simulink model "MuscleGeometry"  (R2024b)
settings: Solver=VariableStepAuto  StartTime=0.0  StopTime=10.0  RelTol=1e-3
undefined symbols (not defined in the file or in its folder): L2, M_BICB, M_BRACH, M_TRIPB
settings Model: Creator=jakub  LastModifiedBy=jakub

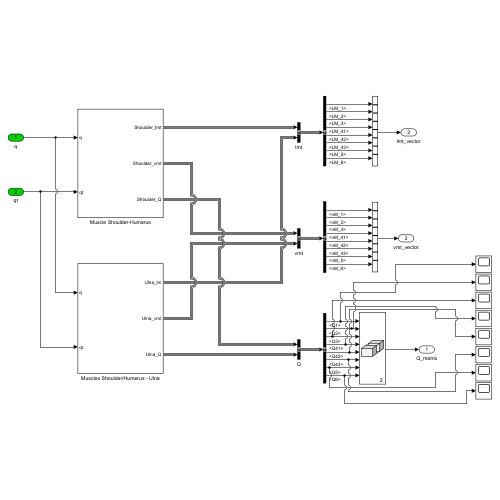
[thumbnail: Simulink's stored preview of the top-level diagram]
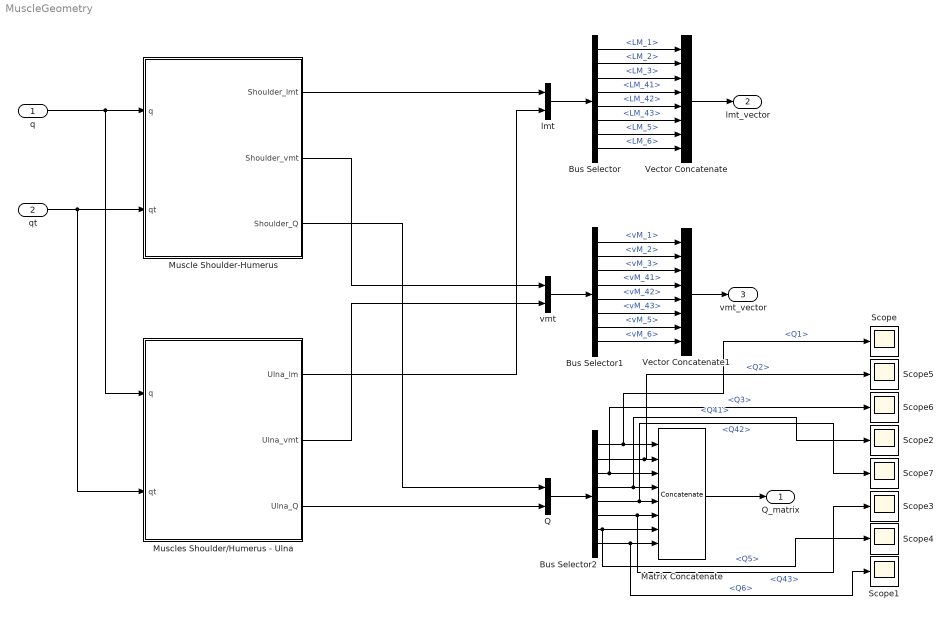
== system MuscleGeometry ==
  q : Inport  OutDataTypeStr=double  Unit=rad  PortDimensions=[2 1]  SampleTime=0
  qt : Inport  Port=2  OutDataTypeStr=double  Unit=rad/sec  PortDimensions=[2 1]  SampleTime=0
  Bus Selector : BusSelector  OutputSignals=signal1.LM_1,signal1.LM_2,signal1.LM_3,signal2.LM_41,signal2.LM_42,signal2.LM_43,signal2.LM_5,signal2.LM_6
  Bus Selector1 : BusSelector  OutputSignals=signal1.vM_1,signal1.vM_2,signal1.vM_3,signal2.vM_41,signal2.vM_42,signal2.vM_43,signal2.vM_5,signal2.vM_6
  Bus Selector2 : BusSelector  OutputSignals=signal1.Q1,signal1.Q2,signal1.Q3,signal2.Q41,signal2.Q42,signal2.Q43,signal2.Q5,signal2.Q6
  Matrix Concatenate : Concatenate  NumInputs=8  Mode=Multidimensional array  ConcatenateDimension=2
  Muscle Shoulder-Humerus : Subsystem
  Muscles Shoulder/Humerus - Ulna : Subsystem
  Q : BusCreator  Inputs=2
  Scope{,1..7} (8 alike) : Scope
  Vector Concatenate : Concatenate  NumInputs=8
  Vector Concatenate1 : Concatenate  NumInputs=8
  lmt : BusCreator  Inputs=2
  vmt : BusCreator  Inputs=2
  Q_matrix : Outport  OutDataTypeStr=double  PortDimensions=[2 8]  SampleTime=0
  lmt_vector : Outport  Port=2  OutDataTypeStr=double  Unit=m  PortDimensions=8  SampleTime=0
  vmt_vector : Outport  Port=3  OutDataTypeStr=double  Unit=m/s  PortDimensions=8  SampleTime=0
  wires:
  q/1 -> Muscle Shoulder-Humerus/1(q), Muscles Shoulder/Humerus - Ulna/1(q)
  qt/1 -> Muscle Shoulder-Humerus/2(qt), Muscles Shoulder/Humerus - Ulna/2(qt)
  Muscle Shoulder-Humerus/1(Shoulder_lmt) -> lmt/1
  Muscles Shoulder/Humerus - Ulna/1(Ulna_lm) -> lmt/2
  Muscle Shoulder-Humerus/2(Shoulder_vmt) -> vmt/1
  Muscles Shoulder/Humerus - Ulna/2(Ulna_vmt) -> vmt/2
  Muscle Shoulder-Humerus/3(Shoulder_Q) -> Q/1
  Muscles Shoulder/Humerus - Ulna/3(Ulna_Q) -> Q/2
  lmt/1 -> Bus Selector/1
  Bus Selector/1 -> Vector Concatenate/1  "<LM_1>"
  Bus Selector/2 -> Vector Concatenate/2  "<LM_2>"
  Bus Selector/3 -> Vector Concatenate/3  "<LM_3>"
  Bus Selector/4 -> Vector Concatenate/4  "<LM_41>"
  Bus Selector/5 -> Vector Concatenate/5  "<LM_42>"
  Bus Selector/6 -> Vector Concatenate/6  "<LM_43>"
  Bus Selector/7 -> Vector Concatenate/7  "<LM_5>"
  Bus Selector/8 -> Vector Concatenate/8  "<LM_6>"
  Vector Concatenate/1 -> lmt_vector/1
  vmt/1 -> Bus Selector1/1
  Bus Selector1/1 -> Vector Concatenate1/1  "<vM_1>"
  Bus Selector1/2 -> Vector Concatenate1/2  "<vM_2>"
  Bus Selector1/3 -> Vector Concatenate1/3  "<vM_3>"
  Bus Selector1/4 -> Vector Concatenate1/4  "<vM_41>"
  Bus Selector1/5 -> Vector Concatenate1/5  "<vM_42>"
  Bus Selector1/6 -> Vector Concatenate1/6  "<vM_43>"
  Bus Selector1/7 -> Vector Concatenate1/7  "<vM_5>"
  Bus Selector1/8 -> Vector Concatenate1/8  "<vM_6>"
  Q/1 -> Bus Selector2/1
  Bus Selector2/1 -> Scope/1, Matrix Concatenate/1  "<Q1>"
  Bus Selector2/2 -> Scope5/1, Matrix Concatenate/2  "<Q2>"
  Bus Selector2/3 -> Scope6/1, Matrix Concatenate/3  "<Q3>"
  Bus Selector2/4 -> Scope2/1, Matrix Concatenate/4  "<Q41>"
  Bus Selector2/5 -> Scope7/1, Matrix Concatenate/5  "<Q42>"
  Bus Selector2/6 -> Scope3/1, Matrix Concatenate/6  "<Q43>"
  Bus Selector2/7 -> Scope4/1, Matrix Concatenate/7  "<Q5>"
  Bus Selector2/8 -> Scope1/1, Matrix Concatenate/8  "<Q6>"
  Vector Concatenate1/1 -> vmt_vector/1
  Matrix Concatenate/1 -> Q_matrix/1

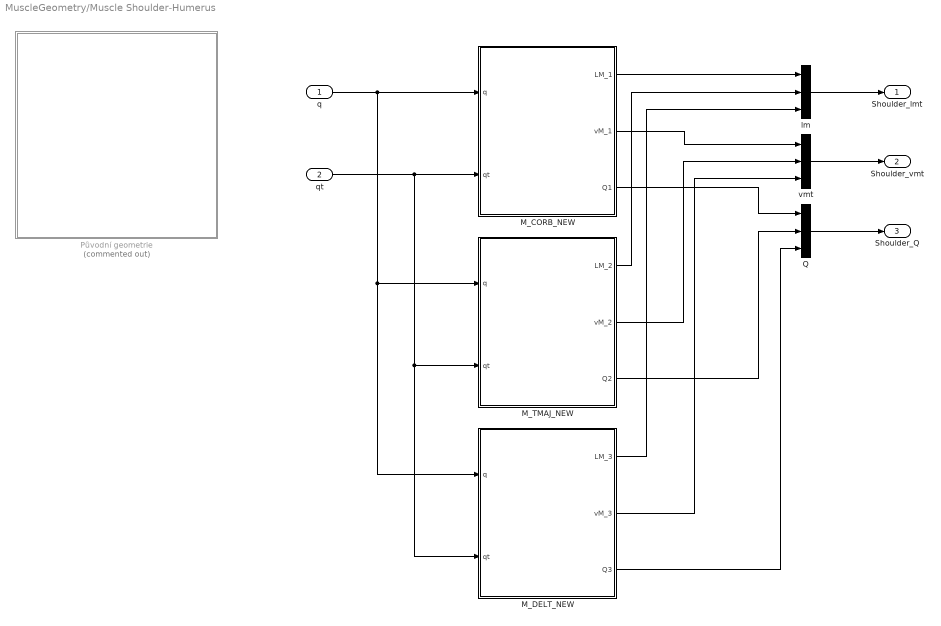
== system MuscleGeometry/Muscle Shoulder-Humerus ==
  q : Inport  OutDataTypeStr=double  Unit=rad  PortDimensions=[2 1]  SampleTime=0
  qt : Inport  Port=2  OutDataTypeStr=double  Unit=rad/sec  PortDimensions=[2 1]  SampleTime=0
  M_CORB_NEW : MATLAB Function  TreatAsAtomicUnit=on
  M_DELT_NEW : MATLAB Function  TreatAsAtomicUnit=on
  M_TMAJ_NEW : MATLAB Function  TreatAsAtomicUnit=on
  Původní geometrie : Subsystem  Commented=on
  Q : BusCreator  Inputs=3
  lm : BusCreator  Inputs=3
  vmt : BusCreator  Inputs=3
  Shoulder_lmt : Outport  OutDataTypeStr=double  Unit=m  PortDimensions=3  SampleTime=0
  Shoulder_vmt : Outport  Port=2  OutDataTypeStr=double  Unit=m/s  PortDimensions=3  SampleTime=0
  Shoulder_Q : Outport  Port=3
  wires:
  M_DELT_NEW/3(Q3) -> Q/3
  M_CORB_NEW/3(Q1) -> Q/1
  lm/1 -> Shoulder_lmt/1
  M_TMAJ_NEW/1(LM_2) -> lm/2
  vmt/1 -> Shoulder_vmt/1
  M_TMAJ_NEW/2(vM_2) -> vmt/2
  M_DELT_NEW/2(vM_3) -> vmt/3
  M_TMAJ_NEW/3(Q2) -> Q/2
  M_CORB_NEW/2(vM_1) -> vmt/1
  M_DELT_NEW/1(LM_3) -> lm/3
  M_CORB_NEW/1(LM_1) -> lm/1
  Q/1 -> Shoulder_Q/1
  qt/1 -> M_DELT_NEW/2(qt), M_TMAJ_NEW/2(qt), M_CORB_NEW/2(qt)
  q/1 -> M_CORB_NEW/1(q), M_DELT_NEW/1(q), M_TMAJ_NEW/1(q)

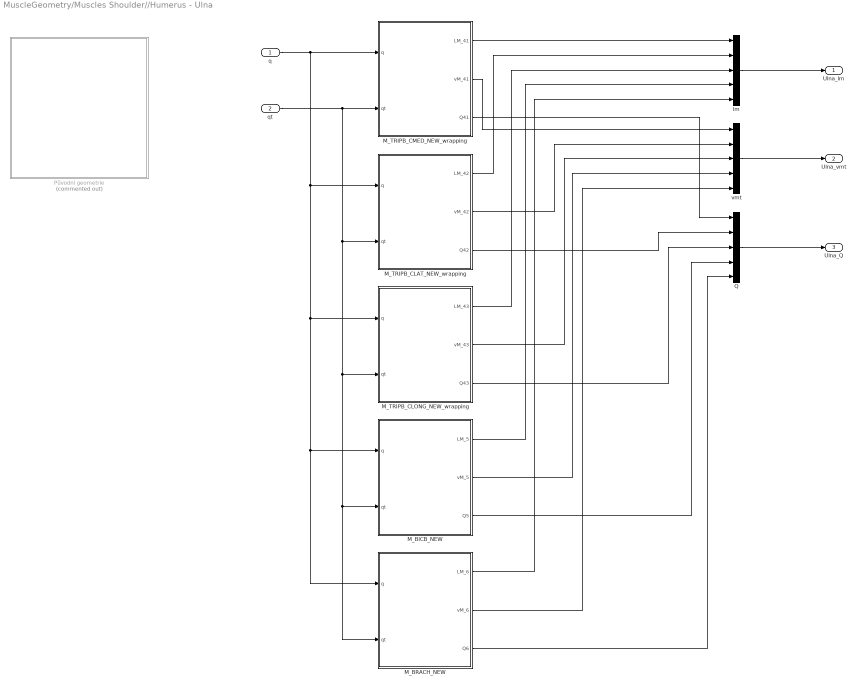
== system MuscleGeometry/Muscles Shoulder//Humerus - Ulna ==
  q : Inport  OutDataTypeStr=double  Unit=rad  PortDimensions=2  SampleTime=0
  qt : Inport  Port=2  OutDataTypeStr=double  Unit=rad/sec  PortDimensions=2  SampleTime=0
  M_BICB_NEW : MATLAB Function  TreatAsAtomicUnit=on
  M_BRACH_NEW : MATLAB Function  TreatAsAtomicUnit=on
  M_TRIPB_CLAT_NEW_wrapping : MATLAB Function  TreatAsAtomicUnit=on
  M_TRIPB_CLONG_NEW_wrapping : MATLAB Function  TreatAsAtomicUnit=on
  M_TRIPB_CMED_NEW_wrapping : MATLAB Function  TreatAsAtomicUnit=on
  Původní geometrie : Subsystem  Commented=on
  Q : BusCreator  Inputs=5
  lm : BusCreator  Inputs=5
  vmt : BusCreator  Inputs=5
  Ulna_lm : Outport
  Ulna_vmt : Outport  Port=2
  Ulna_Q : Outport  Port=3
  wires:
  M_TRIPB_CLAT_NEW_wrapping/1(LM_42) -> lm/2
  M_BRACH_NEW/1(LM_6) -> lm/5
  M_TRIPB_CMED_NEW_wrapping/1(LM_41) -> lm/1
  vmt/1 -> Ulna_vmt/1
  qt/1 -> M_TRIPB_CMED_NEW_wrapping/2(qt), M_BRACH_NEW/2(qt), M_BICB_NEW/2(qt), M_TRIPB_CLONG_NEW_wrapping/2(qt), M_TRIPB_CLAT_NEW_wrapping/2(qt)
  M_TRIPB_CLAT_NEW_wrapping/3(Q42) -> Q/2
  Q/1 -> Ulna_Q/1
  lm/1 -> Ulna_lm/1
  M_TRIPB_CMED_NEW_wrapping/2(vM_41) -> vmt/1
  M_TRIPB_CMED_NEW_wrapping/3(Q41) -> Q/1
  M_TRIPB_CLAT_NEW_wrapping/2(vM_42) -> vmt/2
  M_TRIPB_CLONG_NEW_wrapping/3(Q43) -> Q/3
  M_TRIPB_CLONG_NEW_wrapping/2(vM_43) -> vmt/3
  M_BRACH_NEW/2(vM_6) -> vmt/5
  M_BRACH_NEW/3(Q6) -> Q/5
  M_TRIPB_CLONG_NEW_wrapping/1(LM_43) -> lm/3
  M_BICB_NEW/1(LM_5) -> lm/4
  M_BICB_NEW/2(vM_5) -> vmt/4
  M_BICB_NEW/3(Q5) -> Q/4
  q/1 -> M_TRIPB_CMED_NEW_wrapping/1(q), M_BRACH_NEW/1(q), M_BICB_NEW/1(q), M_TRIPB_CLONG_NEW_wrapping/1(q), M_TRIPB_CLAT_NEW_wrapping/1(q)

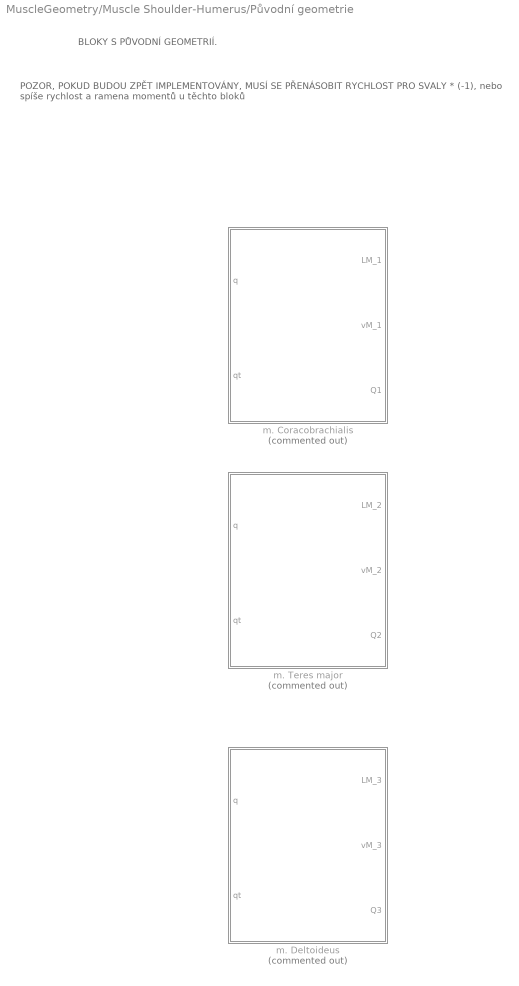
== system MuscleGeometry/Muscle Shoulder-Humerus/Původní geometrie ==
  note: POZOR, POKUD BUDOU ZPĚT IMPLEMENTOVÁNY, MUSÍ SE PŘENÁSOBIT RYCHLOST PRO SVALY * (-1), nebo spíše rychlost a ramena momentů u těchto bloků
  note: BLOKY S PŮVODNÍ GEOMETRIÍ.
  m. Coracobrachialis : MATLAB Function  Commented=on  TreatAsAtomicUnit=on
  m. Deltoideus : MATLAB Function  Commented=on  TreatAsAtomicUnit=on
  m. Teres major : MATLAB Function  Commented=on  TreatAsAtomicUnit=on

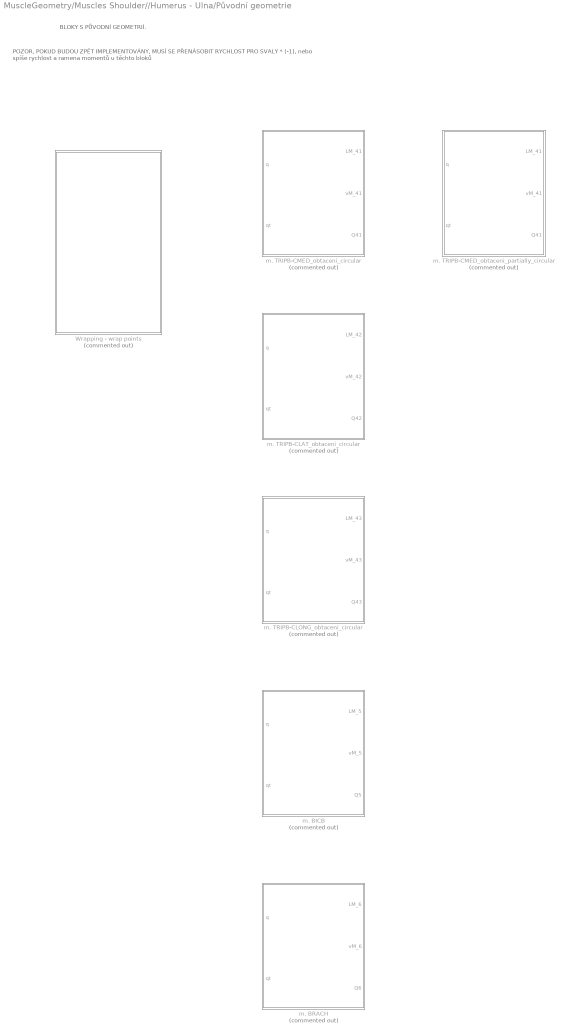
== system MuscleGeometry/Muscles Shoulder//Humerus - Ulna/Původní geometrie ==
  note: BLOKY S PŮVODNÍ GEOMETRIÍ.
  note: POZOR, POKUD BUDOU ZPĚT IMPLEMENTOVÁNY, MUSÍ SE PŘENÁSOBIT RYCHLOST PRO SVALY * (-1), nebo spíše rychlost a ramena momentů u těchto bloků
  Wrapping - wrap points : Subsystem  Commented=on
  m. BICB : MATLAB Function  Commented=on  TreatAsAtomicUnit=on
  m. BRACH : MATLAB Function  Commented=on  TreatAsAtomicUnit=on
  m. TRIPB-CLAT_obtaceni_circular : MATLAB Function  Commented=on  TreatAsAtomicUnit=on
  m. TRIPB-CLONG_obtaceni_circular : MATLAB Function  Commented=on  TreatAsAtomicUnit=on
  m. TRIPB-CMED_obtaceni_circular : MATLAB Function  Commented=on  TreatAsAtomicUnit=on
  m. TRIPB-CMED_obtaceni_partially_circular : MATLAB Function  Commented=on  TreatAsAtomicUnit=on

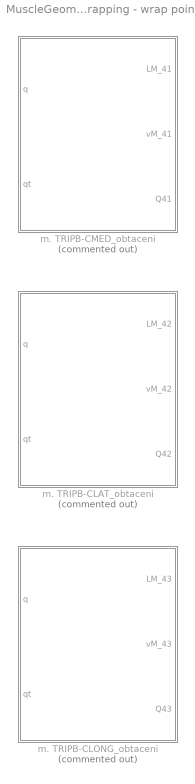
== system MuscleGeometry/Muscles Shoulder//Humerus - Ulna/Původní geometrie/Wrapping - wrap points ==
  m. TRIPB-CLAT_obtaceni : MATLAB Function  Commented=on  TreatAsAtomicUnit=on
  m. TRIPB-CLONG_obtaceni : MATLAB Function  Commented=on  TreatAsAtomicUnit=on
  m. TRIPB-CMED_obtaceni : MATLAB Function  Commented=on  TreatAsAtomicUnit=on

== matlab function MuscleGeometry/Muscles Shoulder//Humerus - Ulna/Původní geometrie/m. BICB ==
  data: LM_5 output double size=1; q input double size=[2 1]; qt input double size=[2 1]; vM_5 output double size=1; M_BICB parameter; Q5 output double size=[2 1]; L2 parameter double size=1
function [LM_5,vM_5, Q5] = MUSCLE_BICB(q,qt,M_BICB, L2)
   
    fi12 = q(1);
    fi12t = qt(1);
    fi13 = q(2);
    fi13t = qt(2);
      
     % Parameters
        % A point in local system "3"
            x3A = M_BICB.x3;
        % B point in local system "1"
            x1B = M_BICB.x1;
            y1B = M_BICB.y1;
    
    % Global coordinates of significant points    
        pA = [L2*cos(fi12) + x3A*cos(fi13);
              L2*sin(fi12) + x3A*sin(fi13)];

        pB = [x1B;
              y1B];

% OUTPUT
    % Muscle geometry
        % Length AB
            LM_5 = norm(pB-pA);

        % Unit vectors
            eAB = (pB-pA)/norm(pB-pA);

        %
            pfi12 = [ -L2*sin(fi12);
                       L2*cos(fi12)];

            pfi13 = [-x3A*sin(fi13);
                      x3A*cos(fi13)];

     % Muscle velocity


        % Final velocity in muscle
            vM_5 = dot(eAB,fi12t*pfi12 + fi13t*pfi13);

    % Vector Q - Generalized forces
        Q_1 = dot(eAB,pfi12);
        Q_2 = dot(eAB,pfi13);

        % Compact form
        Q5 = [Q_1;Q_2];
    
end

== matlab function MuscleGeometry/Muscles Shoulder//Humerus - Ulna/Původní geometrie/m. BRACH ==
  data: LM_6 output double size=1; q input double size=[2 1]; qt input double size=[2 1]; vM_6 output double size=1; M_BRACH parameter; Q6 output double size=[2 1]; L2 parameter double size=1
function [LM_6,vM_6, Q6] = MUSCLE_BRACH(q,qt,M_BRACH, L2)
   
    fi12 = q(1);
    fi12t = qt(1);
    fi13 = q(2);
    fi13t = qt(2);
    
      
     % Parameters
        % A point in local system "3"
            x3A = M_BRACH.x3;
        % B point in local system "2"
            x2B = M_BRACH.x2;

    % Global coordinates of significant points    
        pA = [L2*cos(fi12) + x3A*cos(fi13);
              L2*sin(fi12) + x3A*sin(fi13)];

        pB = [x2B*cos(fi12);
              x2B*sin(fi12)];

% OUTPUT
    % Muscle geometry
        % Length AB
            LM_6 = norm(pB-pA);

        % Unit vectors
            eAB = (pB-pA)/norm(pB-pA);

        %
            pfi12 = [ (-L2+x2B)*sin(fi12);
                       (L2-x2B)*cos(fi12)];

            pfi13 = [-x3A*sin(fi13);
                      x3A*cos(fi13)];

     % Muscle velocity


        % Final velocity in muscle
            vM_6 = dot(eAB,fi12t*pfi12 + fi13t*pfi13);

    % Vector Q - Generalized forces
        Q_1 = dot(eAB,pfi12);
        Q_2 = dot(eAB,pfi13);

        % Compact form
        Q6 = [Q_1;Q_2];
    
end

== matlab function MuscleGeometry/Muscles Shoulder//Humerus - Ulna/M_TRIPB_CMED_NEW_wrapping ==
  data: LM_41 output double size=1; q input double size=[2 1]; qt input double size=[2 1]; vM_41 output double size=1; Q41 output double size=[2 1]
function [LM_41, vM_41, Q41] = MUSCLE_TRIPB_CMED(q, qt)
% VSTUPY:
% q  = [fi12; fi13]         % Úhly
% qt = [fi12_dot; fi13_dot] % Rychlosti úhlů

    % Rozbalení vstupních proměnných
    fi12 = q(1);
    fi13 = q(2);
    fi12_dot = qt(1);
    fi13_dot = qt(2);

    % Přímé volání funkcí
    LM_41 = M_TRIPB_CMED_LM(fi12, fi13);
    vM_41 = M_TRIPB_CMED_vM(fi12, fi13, fi12_dot, fi13_dot);
    Q41 = M_TRIPB_CMED_Q(fi12, fi13);
end

== matlab function MuscleGeometry/Muscle Shoulder-Humerus/M_CORB_NEW ==
  data: LM_1 output double size=1; q input double size=[2 1]; qt input double size=[2 1]; vM_1 output double size=1; Q1 output double size=[2 1]
function [LM_1, vM_1, Q1] = MUSCLE_CORB(q, qt)
% VSTUPY:
% q  = [fi12; fi13]         % Úhly
% qt = [fi12_dot; fi13_dot] % Rychlosti úhlů

    % Rozbalení vstupních proměnných
    fi12 = q(1);
    fi12_dot = qt(1);

    % Přímé volání funkcí
    LM_1 = M_CORB_LM(fi12);
    vM_1 = M_CORB_vM(fi12, fi12_dot);
    Q1 = M_CORB_Q(fi12);
end

== matlab function MuscleGeometry/Muscle Shoulder-Humerus/M_DELT_NEW ==
  data: LM_3 output double size=1; q input double size=[2 1]; qt input double size=[2 1]; vM_3 output double size=1; Q3 output double size=[2 1]
function [LM_3, vM_3, Q3] = MUSCLE_DELT(q, qt)
% VSTUPY:
% q  = [fi12; fi13]         % Úhly
% qt = [fi12_dot; fi13_dot] % Rychlosti úhlů

    % Rozbalení vstupních proměnných
    fi12 = q(1);
    fi12_dot = qt(1);

    % Přímé volání funkcí
    LM_3 = M_DELT_LM(fi12);
    vM_3 = M_DELT_vM(fi12, fi12_dot);
    Q3 = M_DELT_Q(fi12);
end

== matlab function MuscleGeometry/Muscles Shoulder//Humerus - Ulna/Původní geometrie/m. TRIPB-CLAT_obtaceni_circular ==
  data: LM_42 output double size=1; q input double size=[2 1]; qt input double size=[2 1]; vM_42 output double size=1; M_TRIPB parameter; Q42 output double size=[2 1]; L2 parameter double size=1
function [LM_42,vM_42, Q42] = MUSCLE_TRIPB_CLAT(q,qt,M_TRIPB, L2)
   
    fi12 = q(1);
    fi12t = qt(1);
    fi13 = q(2);
    fi13t = qt(2);
      
      % Parameters
        % A point in local system "3"
            x3A = M_TRIPB.CLAT.x3;
            y3A = M_TRIPB.CLAT.y3;
        % B point in local system "2"
            x2B = M_TRIPB.CLAT.x2;
            y2B = M_TRIPB.CLAT.y2;

        % Wrapping points
            % W2 - humerus
                x2W2 = M_TRIPB.CLAT.x2W2;
                y2W2 = M_TRIPB.CLAT.y2W2;
            % W3 - ulna radius
                x3W3 = M_TRIPB.CLAT.x3W3;
                y3W3 = M_TRIPB.CLAT.y3W3;

                
    
    % Global coordinates of significant points    
        pA = [L2*cos(fi12) + x3A*cos(fi13) - y3A*sin(fi13);
              L2*sin(fi12) + x3A*sin(fi13) + y3A*cos(fi13)];

        pW3 = [L2*cos(fi12) + x3W3*cos(fi13) - y3W3*sin(fi13);
               L2*sin(fi12) + x3W3*sin(fi13) + y3W3*cos(fi13)];

        pW2 = [x2W2*cos(fi12) - y2W2*sin(fi12);
               x2W2*sin(fi12) + y2W2*cos(fi12)];

        pB = [x2B*cos(fi12) - y2B*sin(fi12);
              x2B*sin(fi12) + y2B*cos(fi12)];

% OUTPUT
    % Muscle geometry
        % Length AB
            LM_42_straight = norm(pW2-pB) + norm(pW3-pA);
            LM_42_circ = norm(pW3-pW2);
            LM_42 = LM_42_straight + LM_42_circ;

        % Unit vectors
            eAW3 = (pW3-pA)/norm(pW3-pA);
            eW3W2 = (pW2-pW3)/norm(pW2-pW3);
            eBW2 = (pW2-pB)/norm(pW2-pB);

        %
            pAfi12 = [-L2*sin(fi12);
                       L2*cos(fi12)];

            pAfi13 = [-x3A*sin(fi13) - y3A*cos(fi13);
                       x3A*cos(fi13) - y3A*sin(fi13)];

            pW3fi12 = [-L2*sin(fi12);
                        L2*cos(fi12)];

            pW3fi13 = [-x3W3*sin(fi13) - y3W3*cos(fi13);
                        x3W3*cos(fi13) - y3W3*sin(fi13)];

            pW2fi12 = [-x2W2*sin(fi12) - y2W2*cos(fi12);
                        x2W2*cos(fi12) - y2W2*sin(fi12)];
            
            pBfi12 = [-x2B*sin(fi12) - y2B*cos(fi12);
                       x2B*cos(fi12) - y2B*sin(fi12)];

     % Muscle velocity


        % Final velocity in muscle
            vM_42 = dot(eAW3,fi12t*(pAfi12 - pW3fi12) + fi13t*(pAfi13-pW3fi13)) + dot(eW3W2,fi12t*(pW3fi12-pW2fi12) + fi13t*pW3fi13) + dot(eBW2,fi12t*(-pW2fi12 + pBfi12));

    % Vector Q - Generalized forces
        Q_1 = dot(eAW3,pAfi12-pW3fi12) + dot(eW3W2,pW3fi12-pW2fi12) + dot(eBW2,-pW2fi12+pBfi12);
        Q_2 = dot(eAW3,pAfi13-pW3fi13) + dot(eW3W2,pW3fi13);

        % Compact form
        Q42 = [Q_1;Q_2];
end

== matlab function MuscleGeometry/Muscles Shoulder//Humerus - Ulna/Původní geometrie/m. TRIPB-CLONG_obtaceni_circular ==
  data: LM_43 output double size=1; q input double size=[2 1]; qt input double size=[2 1]; vM_43 output double size=1; M_TRIPB parameter; Q43 output double size=[2 1]; L2 parameter double size=1
function [LM_43,vM_43, Q43] = MUSCLE_TRIPB_CLONG(q,qt,M_TRIPB, L2)
   
    fi12 = q(1);
    fi12t = qt(1);
    fi13 = q(2);
    fi13t = qt(2);
      
      % Parameters
        % A point in local system "3"
            x3A = M_TRIPB.CLONG.x3;
            y3A = M_TRIPB.CLONG.y3;
        % B point in local system "1"
            x1B = M_TRIPB.CLONG.x1;
            y1B = M_TRIPB.CLONG.y1;

        % Wrapping
            % W2
                r = M_TRIPB.CLONG.r;
                r1B = M_TRIPB.CLONG.r1B;
                alpha1 = M_TRIPB.CLONG.beta1 + pi/2 + fi12;

                LBE = norm([x1B;y1B] - [L2*cos(fi12);L2*sin(fi12)]);
                beta2 = asin(r1B/LBE*sin(alpha1));
                alpha2 = acos(r/LBE);

                x2W2 = L2 - r*cos(beta2 + alpha2);
                y2W2 = -r*sin(beta2 + alpha2);

            % W3 - ulna radius
                x3W3 = M_TRIPB.CLONG.x3W3;
                y3W3 = M_TRIPB.CLONG.y3W3;
    
    % Global coordinates of significant points    
        pA = [L2*cos(fi12) + x3A*cos(fi13) - y3A*sin(fi13);
              L2*sin(fi12) + x3A*sin(fi13) + y3A*cos(fi13)];

        pW3 = [L2*cos(fi12) + x3W3*cos(fi13) - y3W3*sin(fi13);
               L2*sin(fi12) + x3W3*sin(fi13) + y3W3*cos(fi13)];

        pW2 = [x2W2*cos(fi12) - y2W2*sin(fi12);
               x2W2*sin(fi12) + y2W2*cos(fi12)];

        pB = [x1B;
              y1B];

% OUTPUT
    % Muscle geometry
        % Length AB
            LM_43_straight = norm(pW2-pB) + norm(pW3-pA);
            LM_43_circ = norm(pW3-pW2);
            LM_43 = LM_43_straight + LM_43_circ;

        % Unit vectors
            eAW3 = (pW3-pA)/norm(pW3-pA);
            eW3W2 = (pW2-pW3)/norm(pW2-pW3);
            eBW2 = (pW2-pB)/norm(pW2-pB);

        %
            pAfi12 = [-L2*sin(fi12);
                       L2*cos(fi12)];

            pAfi13 = [-x3A*sin(fi13) - y3A*cos(fi13);
                       x3A*cos(fi13) - y3A*sin(fi13)];

            pW3fi12 = [-L2*sin(fi12);
                        L2*cos(fi12)];

            pW3fi13 = [-x3W3*sin(fi13) - y3W3*cos(fi13);
                        x3W3*cos(fi13) - y3W3*sin(fi13)];

            pW2fi12 = [-x2W2*sin(fi12) - y2W2*cos(fi12);
                        x2W2*cos(fi12) - y2W2*sin(fi12)];
            
            pBfi12 = [0;
                      0];
            

     % Muscle velocity

        % Final velocity in muscle
            vM_43 = dot(eAW3,fi12t*(pAfi12 - pW3fi12) + fi13t*(pAfi13-pW3fi13)) + dot(eW3W2,fi12t*(pW3fi12-pW2fi12) + fi13t*pW3fi13) + dot(eBW2,fi12t*(-pW2fi12 + pBfi12));

    % Vector Q - Generalized forces
        Q_1 = dot(eAW3,pAfi12-pW3fi12) + dot(eW3W2,pW3fi12-pW2fi12) + dot(eBW2,-pW2fi12+pBfi12);
        Q_2 = dot(eAW3,pAfi13-pW3fi13) + dot(eW3W2,pW3fi13);

        % Compact form
        Q43 = [Q_1;Q_2];
end

== matlab function MuscleGeometry/Muscle Shoulder-Humerus/M_TMAJ_NEW ==
  data: LM_2 output double size=1; q input double size=[2 1]; qt input double size=[2 1]; vM_2 output double size=1; Q2 output double size=[2 1]
function [LM_2, vM_2, Q2] = MUSCLE_TMAJ(q, qt)
% VSTUPY:
% q  = [fi12; fi13]         % Úhly
% qt = [fi12_dot; fi13_dot] % Rychlosti úhlů

    % Rozbalení vstupních proměnných
    fi12 = q(1);
    fi12_dot = qt(1);

    % Přímé volání funkcí
    LM_2 = M_TMAJ_LM(fi12);
    vM_2 = M_TMAJ_vM(fi12, fi12_dot);
    Q2 = M_TMAJ_Q(fi12);
end

== matlab function MuscleGeometry/Muscles Shoulder//Humerus - Ulna/Původní geometrie/m. TRIPB-CMED_obtaceni_circular ==
  data: LM_41 output double size=1; q input double size=[2 1]; qt input double size=[2 1]; vM_41 output double size=1; M_TRIPB parameter; Q41 output double size=[2 1]; L2 parameter double size=1
function [LM_41,vM_41, Q41] = MUSCLE_TRIPB_CMED(q,qt,M_TRIPB, L2)
   
    fi12 = q(1);
    fi12t = qt(1);
    fi13 = q(2);
    fi13t = qt(2);
      
     % Parameters
        % A point in local system "3"
            x3A = M_TRIPB.CMED.x3;
            y3A = M_TRIPB.CMED.y3;
        % B point in local system "2"
            x2B = M_TRIPB.CMED.x2;
            y2B = M_TRIPB.CMED.y2;

        % Wrapping points
            r = M_TRIPB.CMED.r;
            % W2 - humerus - vyjádřený v systému "2"
                x2W2 = M_TRIPB.CMED.x2W2;
                y2W2 = M_TRIPB.CMED.y2W2;
                alpha2 = M_TRIPB.CMED.alpha2;
            % W3 - ulna radius - vyjádřený v systému "3"
                x3W3 = M_TRIPB.CMED.x3W3;
                y3W3 = M_TRIPB.CMED.y3W3;
                alpha3 = M_TRIPB.CMED.alpha3;

            % W23 - floating - vyjádřený v systému "2" !!
                alpha23 = fi13 - alpha3 - (fi12 + pi + alpha2);
                alpha23 = mod(alpha23, 2*pi);
                % alpha23 = wrapTo2Pi(alpha23);
                x2W23 = L2 - r*cos(alpha2 + alpha23/2);
                y2W23 = -r*sin(alpha2 + alpha23/2);
                
    
    % Global coordinates of significant points    
        pA = [L2*cos(fi12) + x3A*cos(fi13) - y3A*sin(fi13);
              L2*sin(fi12) + x3A*sin(fi13) + y3A*cos(fi13)];

        pW3 = [L2*cos(fi12) + x3W3*cos(fi13) - y3W3*sin(fi13);
               L2*sin(fi12) + x3W3*sin(fi13) + y3W3*cos(fi13)];

        pW2 = [x2W2*cos(fi12) - y2W2*sin(fi12);
               x2W2*sin(fi12) + y2W2*cos(fi12)];

        pW23 = [x2W23*cos(fi12) - y2W23*sin(fi12);
                x2W23*sin(fi12) + y2W23*cos(fi12)];

        pB = [x2B*cos(fi12) - y2B*sin(fi12);
              x2B*sin(fi12) + y2B*cos(fi12)];

% OUTPUT
    % Muscle geometry
        % Length AB
            LM_41_straight = norm(pW2-pB) + norm(pW3-pA);
            % LM_41_circ = (fi13 - alpha3 - (fi12 + pi + alpha2))*M_TRIPB.HUrad;
            LM_41_circ = norm(pW3-pW23) + norm(pW23-pW2);
            LM_41 = LM_41_straight + LM_41_circ;

        % Unit vectors
            eAW3 = (pW3-pA)/norm(pW3-pA);
            eW3W23 = (pW23-pW3)/norm(pW23-pW3);
            eW23W2 = (pW2-pW23)/norm(pW2-pW23);
            eBW2 = (pW2-pB)/norm(pW2-pB);

        %
            pAfi12 = [-L2*sin(fi12);
                       L2*cos(fi12)];

            pAfi13 = [-x3A*sin(fi13) - y3A*cos(fi13);
                       x3A*cos(fi13) - y3A*sin(fi13)];

            pW3fi12 = [-L2*sin(fi12);
                        L2*cos(fi12)];

            pW3fi13 = [-x3W3*sin(fi13) - y3W3*cos(fi13);
                        x3W3*cos(fi13) - y3W3*sin(fi13)];

            %%%

            pW23fi12 = [-x2W23*sin(fi12) - y2W23*cos(fi12) + cos(fi12)*r*sin(alpha2 + alpha23/2)*(-1) - sin(fi12)*(-r*cos(alpha2 + alpha23/2))*(-1);
                         x2W23*cos(fi12) - y2W23*sin(fi12) + sin(fi12)*r*sin(alpha2 + alpha23/2)*(-1) + cos(fi12)*(-r*cos(alpha2 + alpha23/2))*(-1)];

            pW23fi13 = [ + cos(fi12)*r*sin(alpha2 + alpha23/2)*(+1) - sin(fi12)*(-r*cos(alpha2 + alpha23/2))*(+1);
                         + sin(fi12)*r*sin(alpha2 + alpha23/2)*(+1) + cos(fi12)*(-r*cos(alpha2 + alpha23/2))*(+1)];

            %%%

            pW2fi12 = [-x2W2*sin(fi12) - y2W2*cos(fi12);
                        x2W2*cos(fi12) - y2W2*sin(fi12)];
            
            pBfi12 = [-x2B*sin(fi12) - y2B*cos(fi12);
                       x2B*cos(fi12) - y2B*sin(fi12)];

     % Muscle velocity


        % Final velocity in muscle
            vM_41A = dot(eAW3,fi12t*(pAfi12 - pW3fi12) + fi13t*(pAfi13-pW3fi13));
            vM_41W3 = dot(eW3W23,fi12t*(pW3fi12 - pW23fi12) + fi13t*(pW3fi13-pW23fi13));
            vM_41W23 = dot(eW23W2,fi12t*(pW23fi12 - pW2fi12) + fi13t*(pW23fi13));
            vM_41W2 = dot(eBW2,fi12t*(-pW2fi12 + pBfi12));
            vM_41 = vM_41A + vM_41W3 + vM_41W23 + vM_41W2;

    % Vector Q - Generalized forces
        Q_1 = dot(eAW3, pAfi12-pW3fi12) + dot(eW3W23, pW3fi12-pW23fi12) + dot(eW23W2, pW23fi12-pW2fi12) + dot(eBW2, -pW2fi12+pBfi12);
        Q_2 = dot(eAW3,pAfi13-pW3fi13) + dot(eW3W23,pW3fi13--pW23fi13) + dot(eW23W2,pW23fi13);

        % Compact form
        Q41 = [Q_1;Q_2];
end

== matlab function MuscleGeometry/Muscles Shoulder//Humerus - Ulna/M_TRIPB_CLAT_NEW_wrapping ==
  data: LM_42 output double size=1; q input double size=[2 1]; qt input double size=[2 1]; vM_42 output double size=1; Q42 output double size=[2 1]
function [LM_42, vM_42, Q42] = MUSCLE_TRIPB_CLAT(q, qt)
% VSTUPY:
% q  = [fi12; fi13]         % Úhly
% qt = [fi12_dot; fi13_dot] % Rychlosti úhlů

    % Rozbalení vstupních proměnných
    fi12 = q(1);
    fi13 = q(2);
    fi12_dot = qt(1);
    fi13_dot = qt(2);

    % Přímé volání funkcí
    LM_42 = M_TRIPB_CLAT_LM(fi12, fi13);
    vM_42 = M_TRIPB_CLAT_vM(fi12, fi13, fi12_dot, fi13_dot);
    Q42 = M_TRIPB_CLAT_Q(fi12, fi13);
end

== matlab function MuscleGeometry/Muscles Shoulder//Humerus - Ulna/M_BRACH_NEW ==
  data: LM_6 output double size=1; q input double size=[2 1]; qt input double size=[2 1]; vM_6 output double size=1; Q6 output double size=[2 1]
function [LM_6, vM_6, Q6] = MUSCLE_BRACH(q, qt)
% VSTUPY:
% q  = [fi12; fi13]         % Úhly
% qt = [fi12_dot; fi13_dot] % Rychlosti úhlů

    % Rozbalení vstupních proměnných
    fi12 = q(1);
    fi13 = q(2);
    fi12_dot = qt(1);
    fi13_dot = qt(2);

    % Přímé volání funkcí
    LM_6 = M_BRACH_LM(fi12, fi13);
    vM_6 = M_BRACH_vM(fi12, fi13, fi12_dot, fi13_dot);
    Q6 = M_BRACH_Q(fi12, fi13);
end

== matlab function MuscleGeometry/Muscles Shoulder//Humerus - Ulna/M_TRIPB_CLONG_NEW_wrapping ==
  data: LM_43 output double size=1; q input double size=[2 1]; qt input double size=[2 1]; vM_43 output double size=1; Q43 output double size=[2 1]
function [LM_43, vM_43, Q43] = MUSCLE_TRIPB_CLONG(q, qt)
% VSTUPY:
% q  = [fi12; fi13]         % Úhly
% qt = [fi12_dot; fi13_dot] % Rychlosti úhlů

    % Rozbalení vstupních proměnných
    fi12 = q(1);
    fi13 = q(2);
    fi12_dot = qt(1);
    fi13_dot = qt(2);

    % Přímé volání funkcí
    LM_43 = M_TRIPB_CLONG_LM(fi12, fi13);
    vM_43 = M_TRIPB_CLONG_vM(fi12, fi13, fi12_dot, fi13_dot);
    Q43 = M_TRIPB_CLONG_Q(fi12, fi13);
end

== matlab function MuscleGeometry/Muscles Shoulder//Humerus - Ulna/M_BICB_NEW ==
  data: LM_5 output double size=1; q input double size=[2 1]; qt input double size=[2 1]; vM_5 output double size=1; Q5 output double size=[2 1]
function [LM_5, vM_5, Q5] = MUSCLE_BICB(q, qt)
% VSTUPY:
% q  = [fi12; fi13]         % Úhly
% qt = [fi12_dot; fi13_dot] % Rychlosti úhlů

    % Rozbalení vstupních proměnných
    fi12 = q(1);
    fi13 = q(2);
    fi12_dot = qt(1);
    fi13_dot = qt(2);

    % Přímé volání funkcí
    LM_5 = M_BICB_LM(fi12, fi13);
    vM_5 = M_BICB_vM(fi12, fi13, fi12_dot, fi13_dot);
    Q5 = M_BICB_Q(fi12, fi13);
end

== matlab function MuscleGeometry/Muscle Shoulder-Humerus/Původní geometrie/m. Coracobrachialis ==
  data: LM_1 output double size=1; q input double size=[2 1]; qt input double size=[2 1]; vM_1 output double size=1; M_CORB parameter; Q1 output double size=[2 1]
function [LM_1,vM_1, Q1] = MUSCLE_CORACOBACHIALIS(q,qt,M_CORB)
   
    fi12 = q(1);
    fi12t = qt(1);
      
     % Parameters
        % A point in local system "2"
            x2A = M_CORB.x2A;
        % B point in local system "1"
            x1B = M_CORB.x1B;
            y1B = M_CORB.y1B;
    
    % Global coordinates of significant points
        x1A =  x2A*cos(fi12);
        y1A =  x2A*sin(fi12);
    
        pA = [x1A;y1A];
        pB = [x1B;y1B];

% OUTPUT
    % Muscle geometry
        % Length AD
            LM_1 = norm(pB - pA);

        % Unit vectors
            eAB = (pB-pA)/norm(pB-pA);

        %
            pfi12 = [ - x2A*sin(fi12);
                        x2A*cos(fi12)];
            
            
     % Muscle velocity
        vM_1 = fi12t*dot(eAB,pfi12);

    % Vector Q - Generalized forces
        Q_1 = dot(eAB,pfi12);
        Q_2 = 0;

        % Compact form
        Q1 = [Q_1;Q_2];   
end

== matlab function MuscleGeometry/Muscles Shoulder//Humerus - Ulna/Původní geometrie/Wrapping - wrap points/m. TRIPB-CMED_obtaceni ==
  data: LM_41 output double size=1; q input double size=[2 1]; qt input double size=[2 1]; vM_41 output double size=1; M_TRIPB parameter; Q41 output double size=[2 1]; L2 parameter double size=1
function [LM_41,vM_41, Q41] = MUSCLE_TRIPB_CMED(q,qt,M_TRIPB, L2)
   
    fi12 = q(1);
    fi12t = qt(1);
    fi13 = q(2);
    fi13t = qt(2);
      
     % Parameters
        % A point in local system "3"
            x3A = M_TRIPB.CMED.x3;
            y3A = M_TRIPB.CMED.y3;
        % B point in local system "2"
            x2B = M_TRIPB.CMED.x2;
            y2B = M_TRIPB.CMED.y2;

        % E point in local system "2"
            x2E = M_TRIPB.CMED.x2w;
            y2E = M_TRIPB.CMED.y2w;
    
    % Global coordinates of significant points    
        pA = [L2*cos(fi12) + x3A*cos(fi13) - y3A*sin(fi13);
              L2*sin(fi12) + x3A*sin(fi13) + y3A*cos(fi13)];

        pE = [x2E*cos(fi12) - y2E*sin(fi12);
              x2E*sin(fi12) + y2E*cos(fi12)];

        pB = [x2B*cos(fi12) - y2B*sin(fi12);
              x2B*sin(fi12) + y2B*cos(fi12)];

% OUTPUT
    % Muscle geometry
        % Length AB
            LM_41 = norm(pE-pB) + norm(pE-pA);

        % Unit vectors
            eAE = (pE-pA)/norm(pE-pA);
            eBE = (pE-pB)/norm(pE-pB);

        %
            pAfi12 = [-L2*sin(fi12);
                       L2*cos(fi12)];

            pAfi13 = [-x3A*sin(fi13) - y3A*cos(fi13);
                       x3A*cos(fi13) - y3A*sin(fi13)];

            pEfi12 = [-x2E*sin(fi12) - y2E*cos(fi12);
                       x2E*cos(fi12) - y2E*sin(fi12)];
            
            pBfi12 = [-x2B*sin(fi12) - y2B*cos(fi12);
                       x2B*cos(fi12) - y2B*sin(fi12)];

     % Muscle velocity


        % Final velocity in muscle
            vM_41 = dot(eAE,fi12t*(pAfi12 - pEfi12) + fi13t*pAfi13) + dot(eBE,fi12t*(-pEfi12 + pBfi12));

    % Vector Q - Generalized forces
        Q_1 = dot(eAE,pAfi12-pEfi12) + dot(eBE,-pEfi12+pBfi12);
        Q_2 = dot(eAE,pAfi13);

        % Compact form
        Q41 = [Q_1;Q_2];   
end

== matlab function MuscleGeometry/Muscles Shoulder//Humerus - Ulna/Původní geometrie/Wrapping - wrap points/m. TRIPB-CLAT_obtaceni ==
  data: LM_42 output double size=1; q input double size=[2 1]; qt input double size=[2 1]; vM_42 output double size=1; M_TRIPB parameter; Q42 output double size=[2 1]; L2 parameter double size=1
function [LM_42,vM_42, Q42] = MUSCLE_TRIPB_CLAT(q,qt,M_TRIPB, L2)
   
    fi12 = q(1);
    fi12t = qt(1);
    fi13 = q(2);
    fi13t = qt(2);
      
      % Parameters
        % A point in local system "3"
            x3A = M_TRIPB.CLAT.x3;
            y3A = M_TRIPB.CLAT.y3;
        % B point in local system "2"
            x2B = M_TRIPB.CLAT.x2;
            y2B = M_TRIPB.CLAT.y2;

        % E point in local system "2"
            x2E = M_TRIPB.CLAT.x2w;
            y2E = M_TRIPB.CLAT.y2w;
    
    % Global coordinates of significant points    
        pA = [L2*cos(fi12) + x3A*cos(fi13) - y3A*sin(fi13);
              L2*sin(fi12) + x3A*sin(fi13) + y3A*cos(fi13)];

        pE = [x2E*cos(fi12) - y2E*sin(fi12);
              x2E*sin(fi12) + y2E*cos(fi12)];

        pB = [x2B*cos(fi12) - y2B*sin(fi12);
              x2B*sin(fi12) + y2B*cos(fi12)];

% OUTPUT
    % Muscle geometry
        % Length AB
            LM_42 = norm(pE-pB) + norm(pE-pA);

        % Unit vectors
            eAE = (pE-pA)/norm(pE-pA);
            eBE = (pE-pB)/norm(pE-pB);

        %
            pAfi12 = [-L2*sin(fi12);
                       L2*cos(fi12)];

            pAfi13 = [-x3A*sin(fi13) - y3A*cos(fi13);
                       x3A*cos(fi13) - y3A*sin(fi13)];

            pEfi12 = [-x2E*sin(fi12) - y2E*cos(fi12);
                       x2E*cos(fi12) - y2E*sin(fi12)];
            
            pBfi12 = [-x2B*sin(fi12) - y2B*cos(fi12);
                       x2B*cos(fi12) - y2B*sin(fi12)];

     % Muscle velocity


        % Final velocity in muscle
            vM_42 = dot(eAE,fi12t*(pAfi12 - pEfi12) + fi13t*pAfi13) + dot(eBE,fi12t*(-pEfi12 + pBfi12));

    % Vector Q - Generalized forces
        Q_1 = dot(eAE,pAfi12-pEfi12) + dot(eBE,-pEfi12+pBfi12);
        Q_2 = dot(eAE,pAfi13);

        % Compact form
        Q42 = [Q_1;Q_2];
end

== matlab function MuscleGeometry/Muscle Shoulder-Humerus/Původní geometrie/m. Deltoideus ==
  data: LM_3 output double size=1; vM_3 output double size=1; q input double size=[2 1]; qt input double size=[2 1]; M_DELT parameter; Q3 output double size=[2 1]
function [LM_3,vM_3, Q3] = MUSCLE_DELTOIDEUS(q,qt,M_DELT)
   
    fi12 = q(1);
    fi12t = qt(1);
      
     % Parameters
        % A point in local system "2"
        x2A = M_DELT.x2;
        % B point in local system "1"
        x1B = M_DELT.x1;
        y1B = M_DELT.y1;
    
    % Global coordinates of significant points
        x1A =  x2A*cos(fi12);
        y1A =  x2A*sin(fi12);
    
        pA = [x1A;y1A];
        pB = [x1B;y1B];

% OUTPUT
    % Muscle geometry
        % Length AD
            LM_3 = norm(pB - pA);

        % Unit vectors
            eAB = (pB-pA)/norm(pB-pA);

        %
            pfi12 = [ - x2A*sin(fi12);
                        x2A*cos(fi12)];
            
            
     % Muscle velocity
        vM_3 = fi12t*dot(eAB,pfi12);

    % Vector Q - Generalized forces
        Q_1 = dot(eAB,pfi12);
        Q_2 = 0;

        % Compact form
        Q3 = [Q_1;Q_2];    
end

== matlab function MuscleGeometry/Muscles Shoulder//Humerus - Ulna/Původní geometrie/Wrapping - wrap points/m. TRIPB-CLONG_obtaceni ==
  data: LM_43 output double size=1; q input double size=[2 1]; qt input double size=[2 1]; vM_43 output double size=1; M_TRIPB parameter; Q43 output double size=[2 1]; L2 parameter double size=1
function [LM_43,vM_43, Q43] = MUSCLE_TRIPB_CLONG(q,qt,M_TRIPB, L2)
   
    fi12 = q(1);
    fi12t = qt(1);
    fi13 = q(2);
    fi13t = qt(2);
      
      % Parameters
        % A point in local system "3"
            x3A = M_TRIPB.CLONG.x3;
            y3A = M_TRIPB.CLONG.y3;
        % B point in local system "1"
            x1B = M_TRIPB.CLONG.x1;
            y1B = M_TRIPB.CLONG.y1;

        % E point in local system "2"
            x2E = M_TRIPB.CLONG.x2w;
            y2E = M_TRIPB.CLONG.y2w;
    
    % Global coordinates of significant points    
        pA = [L2*cos(fi12) + x3A*cos(fi13) - y3A*sin(fi13);
              L2*sin(fi12) + x3A*sin(fi13) + y3A*cos(fi13)];

        pE = [x2E*cos(fi12) - y2E*sin(fi12);
              x2E*sin(fi12) + y2E*cos(fi12)];

        pB = [x1B;
              y1B];

% OUTPUT
    % Muscle geometry
        % Length AB
            LM_43 = norm(pE-pB) + norm(pE-pA);

        % Unit vectors
            eAE = (pE-pA)/norm(pE-pA);
            eBE = (pE-pB)/norm(pE-pB);

        %
            pAfi12 = [-L2*sin(fi12);
                       L2*cos(fi12)];

            pAfi13 = [-x3A*sin(fi13) - y3A*cos(fi13);
                       x3A*cos(fi13) - y3A*sin(fi13)];

            pEfi12 = [-x2E*sin(fi12) - y2E*cos(fi12);
                       x2E*cos(fi12) - y2E*sin(fi12)];
            

     % Muscle velocity

        % Final velocity in muscle
            vM_43 = dot(eAE,fi12t*(pAfi12 - pEfi12) + fi13t*pAfi13) + dot(eBE,fi12t*(-pEfi12));

    % Vector Q - Generalized forces
        Q_1 = dot(eAE,pAfi12-pEfi12) + dot(eBE,-pEfi12);
        Q_2 = dot(eAE,pAfi13);

        % Compact form
        Q43 = [Q_1;Q_2];
end

== matlab function MuscleGeometry/Muscle Shoulder-Humerus/Původní geometrie/m. Teres major ==
  data: LM_2 output double size=1; q input double size=[2 1]; qt input double size=[2 1]; vM_2 output double size=1; M_TMAJ parameter; Q2 output double size=[2 1]
function [LM_2,vM_2, Q2] = MUSCLE_TERESMAJOR(q,qt,M_TMAJ)
   
    fi12 = q(1);
    fi12t = qt(1);
      
     % Parameters
        % A point in local system "2"
        x2A = M_TMAJ.x2;
        % B point in local system "1"
        x1B = M_TMAJ.x1; 
        y1B = M_TMAJ.y1; 
    
    % Global coordinates of significant points
        x1A =  x2A*cos(fi12);
        y1A =  x2A*sin(fi12);
    
        pA = [x1A;y1A];
        pB = [x1B;y1B];

% OUTPUT
    % Muscle geometry
        % Length AD
            LM_2 = norm(pB - pA);

        % Unit vectors
            eAB = (pB-pA)/norm(pB-pA);

        %
            pfi12 = [ - x2A*sin(fi12);
                        x2A*cos(fi12)];
            
            
     % Muscle velocity
        vM_2 = fi12t*dot(eAB,pfi12);

    % Vector Q - Generalized forces
        Q_1 = dot(eAB,pfi12);
        Q_2 = 0;

        % Compact form
        Q2 = [Q_1;Q_2];    
end

== matlab function MuscleGeometry/Muscles Shoulder//Humerus - Ulna/Původní geometrie/m. TRIPB-CMED_obtaceni_partially_circular ==
  data: LM_41 output double size=1; q input double size=[2 1]; qt input double size=[2 1]; vM_41 output double size=1; M_TRIPB parameter; Q41 output double size=[2 1]; L2 parameter double size=1
function [LM_41,vM_41, Q41] = MUSCLE_TRIPB_CMED(q,qt,M_TRIPB, L2)
   
    fi12 = q(1);
    fi12t = qt(1);
    fi13 = q(2);
    fi13t = qt(2);
      
     % Parameters
        % A point in local system "3"
            x3A = M_TRIPB.CMED.x3;
            y3A = M_TRIPB.CMED.y3;
        % B point in local system "2"
            x2B = M_TRIPB.CMED.x2;
            y2B = M_TRIPB.CMED.y2;

        % Wrapping points
            % W2 - humerus
                x2W2 = M_TRIPB.CMED.x2W2;
                y2W2 = M_TRIPB.CMED.y2W2;
            % W3 - ulna radius
                x3W3 = M_TRIPB.CMED.x3W3;
                y3W3 = M_TRIPB.CMED.y3W3;

                
    
    % Global coordinates of significant points    
        pA = [L2*cos(fi12) + x3A*cos(fi13) - y3A*sin(fi13);
              L2*sin(fi12) + x3A*sin(fi13) + y3A*cos(fi13)];

        pW3 = [L2*cos(fi12) + x3W3*cos(fi13) - y3W3*sin(fi13);
               L2*sin(fi12) + x3W3*sin(fi13) + y3W3*cos(fi13)];

        pW2 = [x2W2*cos(fi12) - y2W2*sin(fi12);
               x2W2*sin(fi12) + y2W2*cos(fi12)];

        pB = [x2B*cos(fi12) - y2B*sin(fi12);
              x2B*sin(fi12) + y2B*cos(fi12)];

% OUTPUT
    % Muscle geometry
        % Length AB
            LM_41_straight = norm(pW2-pB) + norm(pW3-pA);
            % LM_41_circ = (fi13 - alpha3 - (fi12 + pi + alpha2))*M_TRIPB.HUrad;
            LM_41_circ = norm(pW3-pW2);
            LM_41 = LM_41_straight + LM_41_circ;

        % Unit vectors
            eAW3 = (pW3-pA)/norm(pW3-pA);
            eW3W2 = (pW2-pW3)/norm(pW2-pW3);
            eBW2 = (pW2-pB)/norm(pW2-pB);

        %
            pAfi12 = [-L2*sin(fi12);
                       L2*cos(fi12)];

            pAfi13 = [-x3A*sin(fi13) - y3A*cos(fi13);
                       x3A*cos(fi13) - y3A*sin(fi13)];

            pW3fi12 = [-L2*sin(fi12);
                        L2*cos(fi12)];

            pW3fi13 = [-x3W3*sin(fi13) - y3W3*cos(fi13);
                        x3W3*cos(fi13) - y3W3*sin(fi13)];

            pW2fi12 = [-x2W2*sin(fi12) - y2W2*cos(fi12);
                        x2W2*cos(fi12) - y2W2*sin(fi12)];
            
            pBfi12 = [-x2B*sin(fi12) - y2B*cos(fi12);
                       x2B*cos(fi12) - y2B*sin(fi12)];

     % Muscle velocity


        % Final velocity in muscle
            vM_41 = dot(eAW3,fi12t*(pAfi12 - pW3fi12) + fi13t*(pAfi13-pW3fi13)) + dot(eW3W2,fi12t*(pW3fi12-pW2fi12) + fi13t*pW3fi13) + dot(eBW2,fi12t*(-pW2fi12 + pBfi12));

    % Vector Q - Generalized forces
        Q_1 = dot(eAW3,pAfi12-pW3fi12) + dot(eW3W2,pW3fi12-pW2fi12) + dot(eBW2,-pW2fi12+pBfi12);
        Q_2 = dot(eAW3,pAfi13-pW3fi13) + dot(eW3W2,pW3fi13);

        % Compact form
        Q41 = [Q_1;Q_2];
end
